simulink model "sinusoidal"  (Simulink 7.5)
settings: Solver=ode23tb  StartTime=0.0  StopTime=0.1  MaxStep=1e-5  MinStep=1e-7  RelTol=1e-3
libraries: powerlib x10, simulink x1
settings Model: Creator=nikita  LastModifiedBy=nikita

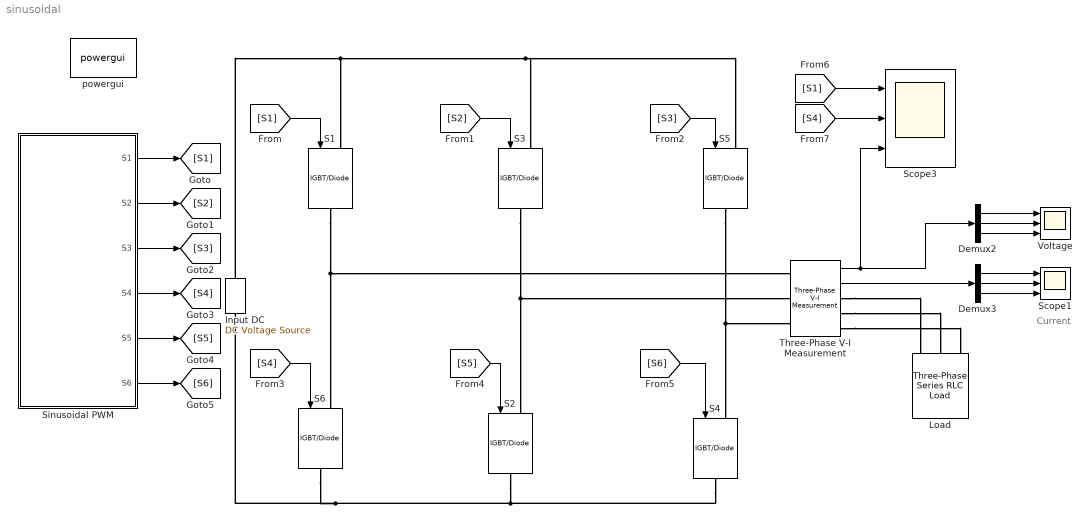
== system sinusoidal ==
  note: Current
  " Load" : powerlib/Elements/Three-Phase Series RLC Load  DialogController=POWERSYS.PowerSysDialog  PhysicalDomain=powersysdomain  SubClassName=unknown  LeftPortType=p1  RightPortType=p1  LConnTagsString=A|B|C  Configuration=Y (grounded)  NominalVoltage=230  NominalFrequency=50  ActivePower=10e3  InductivePower=0  CapacitivePower=0  Measurements=None
  Demux2 : Demux  Outputs=3
  Demux3 : Demux  Outputs=3
  "Input DC " : powerlib/Electrical Sources/DC Voltage Source  DialogController=POWERSYS.PowerSysDialog  SystemSampleTime=-1  Amplitude=350  Measurements=None
  S{1..6} (6 alike) : powerlib/Power Electronics/IGBT//Diode  DialogController=POWERSYS.PowerSysDialog  SystemSampleTime=-1  Ron=1e-3  Rs=1e5  Cs=inf  Measurements=off
  Scope1 : Scope  NumInputPorts=3
      settings: YMin=-100~-100~-100  YMax=100~100~100
  Scope3 : Scope  NumInputPorts=3
      settings: YMin=-5~-5~-400  YMax=5~5~400  SaveName=sinusoidalPWM
  Sinusoidal PWM : Subsystem
  Three-Phase V-I Measurement : powerlib/Measurements/Three-Phase V-I Measurement  DialogController=POWERSYS.PowerSysDialog  SystemSampleTime=-1  VoltageMeasurement=phase-to-phase  SetLabelV=off  LabelV=Vabc  Vpu=off  VpuLL=off  CurrentMeasurement=yes  SetLabelI=off  LabelI=Iabc  Ipu=off  Pbase=100e6  Vbase=500e3  OutputType=Complex  PhasorSimulation=off  PSBequivalent=0
      link override Model/VI/Ia: GotoTag=LibraryTag_Ia
      link override Model/VI/Ib: GotoTag=LibraryTag_Ib
      link override Model/VI/Ic: GotoTag=LibraryTag_Ic
      link override Model/VI/Va: GotoTag=LibraryTag_Va
      link override Model/VI/Vb: GotoTag=LibraryTag_Vb
      link override Model/VI/Vc: GotoTag=LibraryTag_Vc
  Voltage : Scope  NumInputPorts=3
      settings: YMin=-500~-500~-500  YMax=500~500~500  SaveName=SPWMV
  powergui : powerlib/powergui  Priority=1  SystemSampleTime=-1  SimulationMode=Discrete  SampleTime=50e-6  frequency=60  SPID=off  DisableSnubberDevices=off  DisableRonSwitches=off  DisableVfSwitches=off  SwTol=0  Interpol=off  frequencyindice=0  echomessages=off  HookPort=off  DisplayEquations=off  FunctionMessages=off  EnableUseOfTLC=off  x0status=blocks  RestoreLinks=warning  ResistiveCurrentMeasurement=off  Ylog=off  Xlog=on  ShowGrid=off  save=off  variable=ZData  structure=SPWMV  ZoomFFT=off  StartTime=0.0  cycles=2  DisplayStyle=2  fundamental=50  FreqAxis=off  MaxFrequency=1000  frequencyindicesteady=1  display=off  methode=off
  wires:
  Three-Phase V-I Measurement/1 -> Demux2/1, Scope3/3
  Demux2/1 -> Voltage/1
  Demux2/2 -> Voltage/2
  Demux2/3 -> Voltage/3
  Demux3/1 -> Scope1/1
  Demux3/2 -> Scope1/2
  Demux3/3 -> Scope1/3
  Three-Phase V-I Measurement/2 -> Demux3/1
  Sinusoidal PWM/1(S1) -> [S1]
  Sinusoidal PWM/2(S2) -> [S2]
  Sinusoidal PWM/3(S3) -> [S3]
  Sinusoidal PWM/4(S4) -> [S4]
  Sinusoidal PWM/5(S5) -> [S5]
  Sinusoidal PWM/6(S6) -> [S6]
  [S1] -> S1/1
  [S2] -> S3/1
  [S3] -> S5/1
  [S4] -> S6/1
  [S5] -> S2/1
  [S6] -> S4/1
  [S4] -> Scope3/2
  [S1] -> Scope3/1
  connections:
  S4/RConn1 -- S6/RConn1 -- "Input DC "/LConn1 -- S2/RConn1
  S1/RConn1 -- S6/LConn1 -- Three-Phase V-I Measurement/LConn1
  S3/RConn1 -- S2/LConn1 -- Three-Phase V-I Measurement/LConn2
  S5/RConn1 -- S4/LConn1 -- Three-Phase V-I Measurement/LConn3
  Three-Phase V-I Measurement/RConn1 -- " Load"/LConn1
  Three-Phase V-I Measurement/RConn2 -- " Load"/LConn2
  Three-Phase V-I Measurement/RConn3 -- " Load"/LConn3
  "Input DC "/RConn1 -- S5/LConn1 -- S3/LConn1 -- S1/LConn1

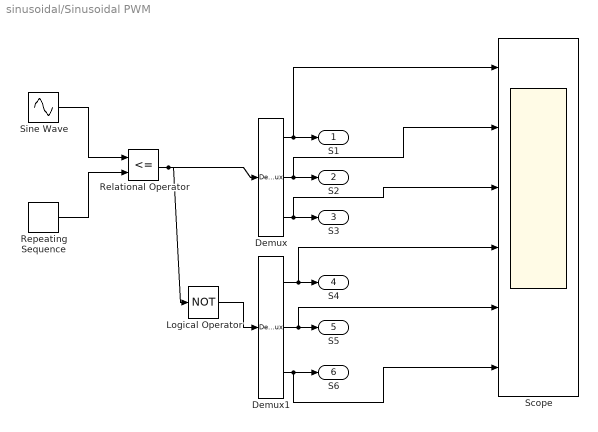
== system sinusoidal/Sinusoidal PWM ==
  Demux : Demux  Outputs=3
  Demux1 : Demux  Outputs=3
  Logical Operator : Logic  Operator=NOT  AllPortsSameDT=off  OutDataTypeMode=boolean  LogicDataType=fixdt(0, 8)  OutDataTypeStr=boolean
  Relational Operator : RelationalOperator  Operator=<=  LogicOutDataTypeMode=boolean  LogicDataType=fixdt(0, 8)  OutDataTypeStr=boolean
  Repeating Sequence : simulink/Sources/Repeating Sequence  SystemSampleTime=-1  rep_seq_t=[0 0.25 0.5 0.75 1]/980  rep_seq_y=[0 1 0 -1 0]
  Scope : Scope  NumInputPorts=6
      settings: YMin=-2~-2~-2~-2~-2~-2  YMax=2~2~2~2~2~2  SaveName=SPWM
  Sine Wave : Sin  Amplitude=[0.8 0.8 0.8]  Bias=0  Frequency=2*pi*50  Phase=[0 2*pi/3 4*pi/3]  Samples=10  SampleTime=0  Offset=0
  S1 : Outport
  S2 : Outport  Port=2  OutDataType=fixdt(1, 16)  OutScaling=2^0
  S3 : Outport  Port=3  OutDataType=fixdt(1, 16)  OutScaling=2^0
  S4 : Outport  Port=4  OutDataType=fixdt(1, 16)  OutScaling=2^0
  S5 : Outport  Port=5  OutDataType=fixdt(1, 16)  OutScaling=2^0
  S6 : Outport  Port=6  OutDataType=fixdt(1, 16)  OutScaling=2^0
  wires:
  Sine Wave/1 -> Relational Operator/1
  Repeating Sequence/1 -> Relational Operator/2
  Relational Operator/1 -> Logical Operator/1, Demux/1
  Logical Operator/1 -> Demux1/1
  Demux/1 -> S1/1, Scope/1
  Demux/2 -> S2/1, Scope/2
  Demux/3 -> S3/1, Scope/3
  Demux1/1 -> S4/1, Scope/4
  Demux1/2 -> S5/1, Scope/5
  Demux1/3 -> S6/1, Scope/6
